simulink model "SimCellule"  (R2014a)
settings: Solver=ode23tb  StartTime=0.0  StopTime=1  FixedStep=11e-6  RelTol=1e-6
values from neighbouring files (symbols this model uses):
  rev_current = flipud(current)    [Init_panneau.m]
  rev_voltage = flipud(voltage)    [Init_panneau.m]
libraries: powerlib x8
settings Model: Creator=hfortin  LastModifiedBy=hugo
settings DataIOCC: SignalLoggingSaveFormat=ModelDataLogs  Refine=4
settings OptimizationCC: ExpressionDepthLimit=2147483647
settings DebuggingCC: UnderspecifiedInitializationDetection=Classic  FcnCallInpInsideContextMsg=UseLocalSettings  StateNameClashWarn=warning
settings GRTTargetCC: CombineOutputUpdateFcns=off  GRTInterface=on

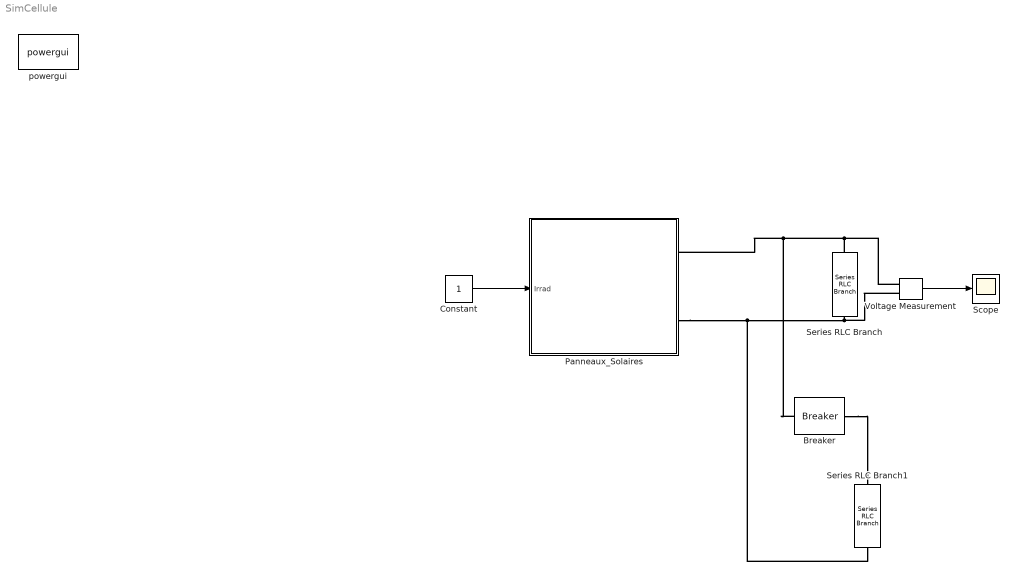
== system SimCellule ==
  Breaker : powerlib/Elements/Breaker  InitialState=0  SwitchingTimes=[1/2]  External=off  BreakerResistance=0.01  SnubberResistance=1e6  SnubberCapacitance=inf  Measurements=None  MoreParameters=on  NoBreakLoop=off
  Constant : Constant
  Panneaux_Solaires : Subsystem
  Scope : Scope
  Series RLC Branch : powerlib/Elements/Series RLC Branch  LConnTagsString=__new0  RConnTagsString=__new0  BranchType=R  Resistance=1000  Inductance=1e-3  SetiL0=off  InitialCurrent=0  Capacitance=1e-6  Setx0=off  InitialVoltage=0  Measurements=None
  Series RLC Branch1 : powerlib/Elements/Series RLC Branch  LConnTagsString=__new0  RConnTagsString=__new0  BranchType=R  Resistance=50  Inductance=1e-3  SetiL0=off  InitialCurrent=0  Capacitance=1e-6  Setx0=off  InitialVoltage=0  Measurements=None
  Voltage Measurement : powerlib/Measurements/Voltage Measurement  PhasorSimulation=off  OutputType=Complex  PSBequivalent=0
  powergui : powerlib/powergui  Priority=1  SimulationMode=Continuous  SolverType=Tustin  SampleTime=11e-6  frequency=60  SPID=off  DisableSnubberDevices=off  DisableRonSwitches=off  DisableVfSwitches=off  SwTol=0  Interpol=off  DisplayEquations=off  Ts=0  methode=off  frequencyindice=0  Pbase=100e6  ErrMax=1e-4  Iterations=50  UnitsV=kV  UnitsW=MW  FunctionMessages=off  echomessages=off  HookPort=off  EnableUseOfTLC=off  x0status=blocks  RestoreLinks=warning  ResistiveCurrentMeasurement=off  Frange=[0:2:500]  Ylog=off  Xlog=on  ShowGrid=off  save=off  variable=ZData  structure=0  ZoomFFT=on  StartTime=0.0  cycles=1  DisplayStyle=1  fundamental=60  FreqAxis=off  MaxFrequency=1000  frequencyindicesteady=1  RmsSteady=1  display=off
  wires:
  Constant/1 -> Panneaux_Solaires/1(Irrad)
  Voltage Measurement/1 -> Scope/1
  connections:
  Panneaux_Solaires/RConn2 -- Series RLC Branch1/RConn1 -- Voltage Measurement/LConn2 -- Series RLC Branch/RConn1
  Series RLC Branch/LConn1 -- Breaker/LConn1 -- Panneaux_Solaires/RConn1 -- Voltage Measurement/LConn1
  Breaker/RConn1 -- Series RLC Branch1/LConn1

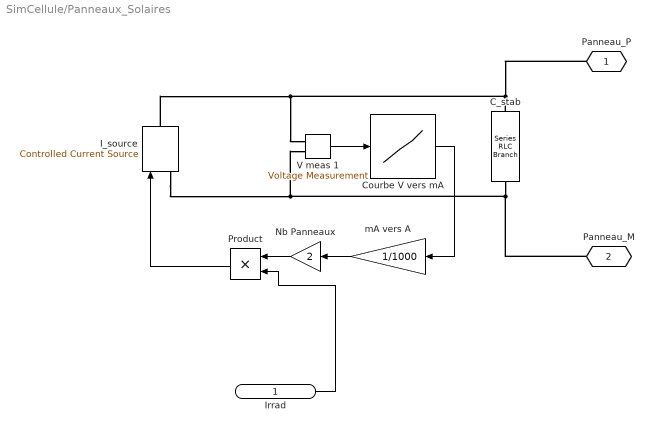
== system SimCellule/Panneaux_Solaires ==
  Irrad : Inport
  C_stab : powerlib/Elements/Series RLC Branch  LConnTagsString=__new0  RConnTagsString=__new0  BranchType=C  Resistance=1  Inductance=1e-3  SetiL0=off  InitialCurrent=0  Capacitance=1e-9  Setx0=off  InitialVoltage=1  Measurements=None
  Courbe V vers mA : Lookup_n-D  NumberOfTableDimensions=1  BreakpointsForDimension1=rev_voltage  Table=rev_current  UseLastTableValue=on  InternalRulePriority=Speed  RndMeth=Simplest  InputSameDT=on
  I_source : powerlib/Electrical Sources/Controlled Current Source  Initialize=off  Source_Type=DC  Amplitude=0  Phase=0  Frequency=0  Measurements=None
  Nb Panneaux : Gain  Gain=2
  Product : Product
  V meas 1 : powerlib/Measurements/Voltage Measurement  PhasorSimulation=off  OutputType=Complex  PSBequivalent=0
  mA vers A : Gain  Gain=1/1000
  Panneau_P : PMIOPort  Port=1  Side=Right
  Panneau_M : PMIOPort  Port=2  Side=Right
  wires:
  Courbe V vers mA/1 -> mA vers A/1
  mA vers A/1 -> Nb Panneaux/1
  V meas 1/1 -> Courbe V vers mA/1
  Nb Panneaux/1 -> Product/1
  Product/1 -> I_source/1
  Irrad/1 -> Product/2
  connections:
  C_stab/RConn1 -- Panneau_M/RConn1 -- I_source/LConn1 -- V meas 1/LConn2
  V meas 1/LConn1 -- Panneau_P/RConn1 -- C_stab/LConn1 -- I_source/RConn1
